simulink model "IP_TEST_PCI6221_2015a"  (R2015a)
settings: Solver=ode3  StartTime=0.0  StopTime=200  RelTol=1e-3
undefined symbols (not defined in the file or in its folder): National_Instruments, PCI
libraries: sldrtlib x3, simulink x1
settings Model: SimulationMode=external  CovHtmlReporting=off  ExtModeTrigDuration=100000  Creator=Alunos  LastModifiedBy=Tomas Teixeira
settings HardwareCC: ProdIntDivRoundTo=Zero  ProdEndianess=LittleEndian  ProdHWDeviceType=Intel->x86/Pentium  TargetIntDivRoundTo=Zero  TargetEndianess=LittleEndian  TargetHWDeviceType=Intel->x86/Pentium
settings RTWCC: SystemTargetFile=rtwin.tlc  TemplateMakefile=rtwin.tmf  Description=Simulink Desktop Real-Time  RTWCompilerOptimization=on
settings CodeAppCC: MaxIdLength=95
settings GRTTargetCC: TargetLangStandard=C99 (ISO)
settings RTWinTargetCC: TargetPreCompLibLocation=C:\Program Files\MATLAB\R2015a\toolbox\sldrt\lib\win32  UseToolchainInfoCompliant=off

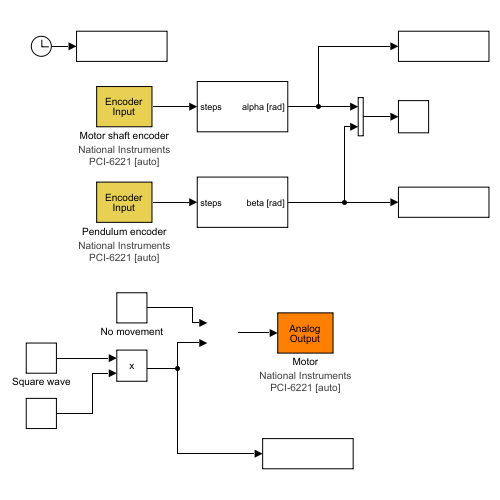
[thumbnail: Simulink's stored preview of the top-level diagram]
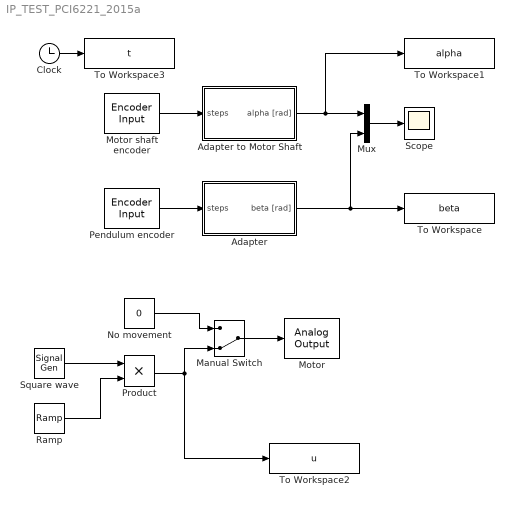
== system IP_TEST_PCI6221_2015a ==
  Adapter : Subsystem
  Adapter to Motor Shaft : Subsystem
  Clock : Clock
  Manual Switch : ManualSwitch  CurrentSetting=0
  Motor : sldrtlib/Analog Output  SampleTime=0.01  MaxMissedTicks=10  ShowMissedTicks=off  YieldWhenWaiting=off  DrvName=National_Instruments/PCI-6221  DrvAddress=4294967295  DrvOptions=[0 0 0 2 2]  Channels=1  RangeMode=1  VoltRange=1  InitialValue=0  FinalValue=0
      settings: AttributesFormatString=National Instruments\nPCI-6221 [auto]
  Motor shaft encoder : sldrtlib/Encoder Input  SampleTime=0.01  MaxMissedTicks=inf  ShowMissedTicks=off  YieldWhenWaiting=off  DrvName=National_Instruments/PCI-6221  DrvAddress=4294967295  DrvOptions=[0 0 0 2 2]  Channels=1  QuadMode=3  IndexPulse=2  InputFilter=Inf  DataType=1
      settings: AttributesFormatString=National Instruments\nPCI-6221 [auto]
  Mux : Mux  Inputs=2
  No movement : Constant  Value=0
  Pendulum encoder : sldrtlib/Encoder Input  SampleTime=0.01  MaxMissedTicks=inf  ShowMissedTicks=off  YieldWhenWaiting=off  DrvName=National_Instruments/PCI-6221  DrvAddress=4294967295  DrvOptions=[0 0 0 2 2]  Channels=2  QuadMode=3  IndexPulse=2  InputFilter=Inf  DataType=1
      settings: AttributesFormatString=National Instruments\nPCI-6221 [auto]
  Product : Product
  Ramp : simulink/Sources/Ramp  slope=1  start=0  X0=0
  Scope : Scope
      settings: TimeRange=Auto  MaxDataPoints=5000  SaveToWorkspace=off  YMin=-3.5  YMax=3.5  SampleTime=-1  DataFormat=Array
  Square wave : SignalGenerator  WaveForm=square  Frequency=.25
  To Workspace : ToWorkspace  VariableName=beta  SaveFormat=Structure With Time  SampleTime=-1
  To Workspace1 : ToWorkspace  VariableName=alpha  SaveFormat=Structure With Time  SampleTime=-1
  To Workspace2 : ToWorkspace  VariableName=u  SaveFormat=Structure With Time  SampleTime=-1
  To Workspace3 : ToWorkspace  VariableName=t  SaveFormat=Timeseries  SampleTime=-1
  wires:
  Mux/1 -> Scope/1
  Manual Switch/1 -> Motor/1
  No movement/1 -> Manual Switch/1
  Pendulum encoder/1 -> Adapter/1(steps)
  Adapter/1(beta [rad]) -> To Workspace/1, Mux/2
  Motor shaft encoder/1 -> Adapter to Motor Shaft/1(steps)
  Adapter to Motor Shaft/1(alpha [rad]) -> To Workspace1/1, Mux/1
  Square wave/1 -> Product/1
  Product/1 -> To Workspace2/1, Manual Switch/2
  Ramp/1 -> Product/2
  Clock/1 -> To Workspace3/1

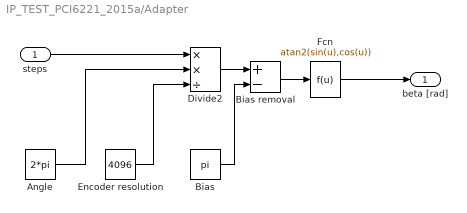
== system IP_TEST_PCI6221_2015a/Adapter ==
  steps : Inport
  Angle : Constant  Value=2*pi
  Bias : Constant  Value=pi
  Bias removal : Sum  Inputs=+-
  Divide2 : Product  Inputs=**/
  Encoder resolution : Constant  Value=4096
  Fcn : Fcn  Expr=atan2(sin(u),cos(u))
  beta [rad] : Outport
  wires:
  Angle/1 -> Divide2/2
  Encoder resolution/1 -> Divide2/3
  steps/1 -> Divide2/1
  Bias removal/1 -> Fcn/1
  Bias/1 -> Bias removal/2
  Divide2/1 -> Bias removal/1
  Fcn/1 -> beta [rad]/1

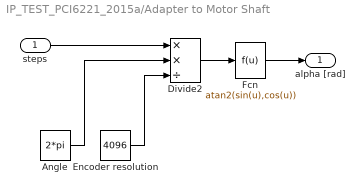
== system IP_TEST_PCI6221_2015a/Adapter to Motor Shaft ==
  steps : Inport
  Angle : Constant  Value=2*pi
  Divide2 : Product  Inputs=**/
  Encoder resolution : Constant  Value=4096
  Fcn : Fcn  Expr=atan2(sin(u),cos(u))
  alpha [rad] : Outport
  wires:
  Angle/1 -> Divide2/2
  Encoder resolution/1 -> Divide2/3
  steps/1 -> Divide2/1
  Divide2/1 -> Fcn/1
  Fcn/1 -> alpha [rad]/1
